simulink model "sldemo_foreach_tiled"  (R2019b)
settings: Solver=FixedStepDiscrete  StartTime=0.0  StopTime=1.0  FixedStep=0.2  RelTol=1e-3  EnableMultiTasking=on
settings Model: Creator=The MathWorks, Inc.  LastModifiedBy=bhisma
settings DataIOCC: LimitDataPoints=on  SaveFormat=Structure
settings OptimizationCC: ExpressionDepthLimit=2147483647  LifeSpan=1  EfficientTunableParamExpr=on
settings DebuggingCC: SolverPrmCheckMsg=warning  FcnCallInpInsideContextMsg=warning  AllowSymbolicDim=off  StateNameClashWarn=warning  SFUnexpectedBacktrackingDiag=warning  SFNoUnconditionalDefaultTransitionDiag=warning  SFExecutionAtInitializationDiag=none  ArithmeticOperatorsInVariantConditions=warning
settings HardwareCC: ProdBitPerPointer=32  ProdBitPerSizeT=32  ProdBitPerPtrDiffT=32  ProdLargestAtomicFloat=None  ProdIntDivRoundTo=Undefined  ProdEndianess=Unspecified  ProdWordSize=32  ProdHWDeviceType=32-bit Generic
settings ModelReferenceCC: PropagateSignalLabelsOutOfModel=off
settings SFSimCC: SimUseLocalCustomCode=off  MATLABDynamicMemAlloc=off  CustomCodeUndefinedFunction=UseInterfaceOnly
settings RTWCC: Description=Real-Time Workshop Embedded Coder  SystemTargetFile=ert.tlc  TemplateMakefile=ert_default_tmf  GenerateReport=on  RTWUseLocalCustomCode=off  IncludeHyperlinkInReport=on  LaunchReport=on
settings CodeAppCC: IgnoreCustomStorageClasses=off  CustomSymbolStrType=$N$R$M  StateflowObjectComments=on  InternalIdentifier=Classic
settings ERTTargetCC: MultiwordLength=2048  GenerateSampleERTMain=on  MatFileLogging=on  SupportVariableSizeSignals=on  ERTCustomFileTemplate=example_file_process.tlc  ConvertIfToSwitch=off  SuppressUnreachableDefaultCases=off
settings ConfigComp: CovMetricSettings=dw  CovHtmlReporting=on  CovSaveCumulativeToWorkspaceVar=on  CovSaveSingleToWorkspaceVar=on  CovExternalEMLEnable=off

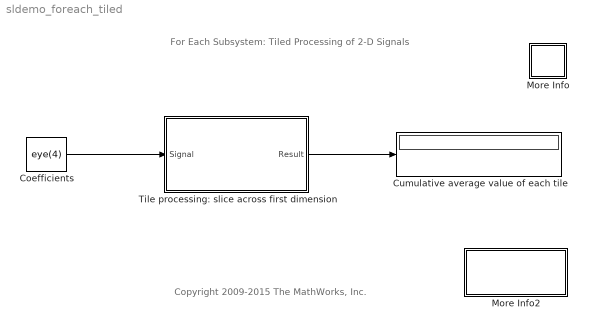
== system sldemo_foreach_tiled ==
  note: Copyright 2009-2015 The MathWorks, Inc.
  note: For Each Subsystem:
      | Tiled Processing of 2-D Signals
  Coefficients : Constant  Value=eye(4)
  Cumulative average value of each tile : Display
  More Info : Subsystem
      settings: OpenFcn=showdemo(bdroot(gcb))
      mask Display: disp('?')
  More Info2 : Subsystem
      settings: OpenFcn=sldemo_foreach_repeat_tile
      mask Display: disp('Double-Click for\nTile Repetition\nImplementation')
  Tile processing: slice across first dimension : Subsystem  TreatAsAtomicUnit=on
      settings: RTWFcnNameOpts=Use subsystem name  RTWFileNameOpts=Use function name
  wires:
  Coefficients/1 -> Tile processing: slice across first dimension/1(Signal)
  Tile processing: slice across first dimension/1(Result) -> Cumulative average value of each tile/1

== system sldemo_foreach_tiled/More Info ==
  note: Bus Block Demonstration
  note: This demonstration shows how signals may be grouped and ungrouped while
      | retaining their names.  In this demonstration, 5 signals are created and labeled
      | appropriately.  These signals are then mux'd together to create a bus of signals.
      | This bus of signals is then fed into the Bus Selector block.  Inside of the Bus
      | Selector block, the Pulse and Chirp signals are chosen to be output from the
      | original signal bus.
      |
      | It is possible to place a nest signal buses and then still retrieve the original signal
      | with its label.

== system sldemo_foreach_tiled/More Info2 ==

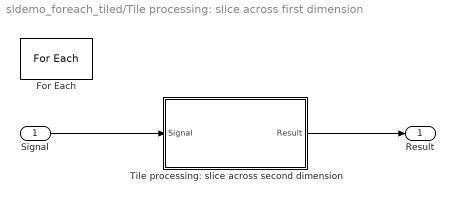
== system sldemo_foreach_tiled/Tile processing: slice across first dimension ==
  Signal : Inport  Partition=on  PartitionDimension=1  PartitionWidth=2  PartitionOffset=0
  For Each : ForEach
  Tile processing: slice across second dimension : Subsystem  TreatAsAtomicUnit=on
      settings: RTWFcnNameOpts=Use subsystem name  RTWFileNameOpts=Use function name
  Result : Outport  ConcatenationDimension=1  VectorParamsAs1DForOutWhenUnconnected=off
  wires:
  Signal/1 -> Tile processing: slice across second dimension/1(Signal)
  Tile processing: slice across second dimension/1(Result) -> Result/1

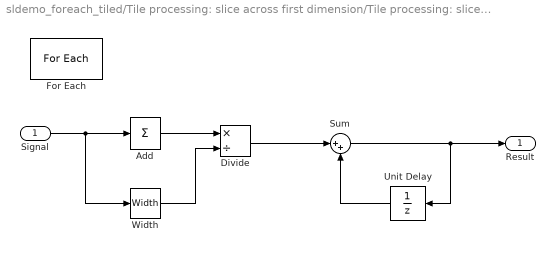
== system sldemo_foreach_tiled/Tile processing: slice across first dimension/Tile processing: slice across second dimension ==
  Signal : Inport  Partition=on  PartitionDimension=2  PartitionWidth=2  PartitionOffset=0
  Add : Sum  Inputs=+
  Divide : Product  Inputs=*/
  For Each : ForEach
  Sum : Sum  Inputs=|++
  Unit Delay : UnitDelay  SampleTime=-1  HasFrameUpgradeWarning=on
  Width : Width
  Result : Outport  ConcatenationDimension=2  VectorParamsAs1DForOutWhenUnconnected=off
  wires:
  Signal/1 -> Add/1, Width/1
  Add/1 -> Divide/1
  Width/1 -> Divide/2
  Divide/1 -> Sum/1
  Sum/1 -> Result/1, Unit Delay/1
  Unit Delay/1 -> Sum/2
